simulink model "anti_windup_cliping_back_calculation"  (R2022b)
settings: Solver=FixedStepAuto  StartTime=0.0  StopTime=200  FixedStep=0.001  RelTol=1e-3
libraries: simulink x2
settings Model: Creator=mrxmi  LastModifiedBy=mrxmi

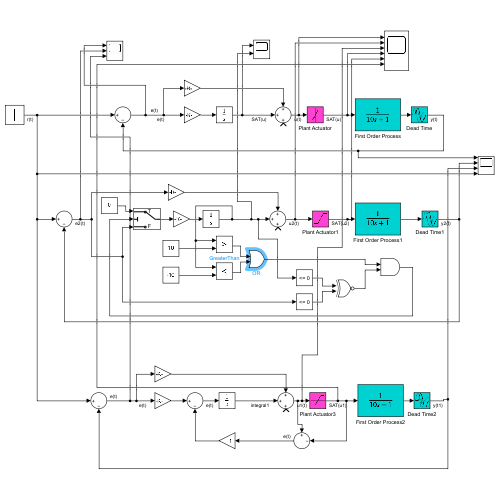
[thumbnail: Simulink's stored preview of the top-level diagram]
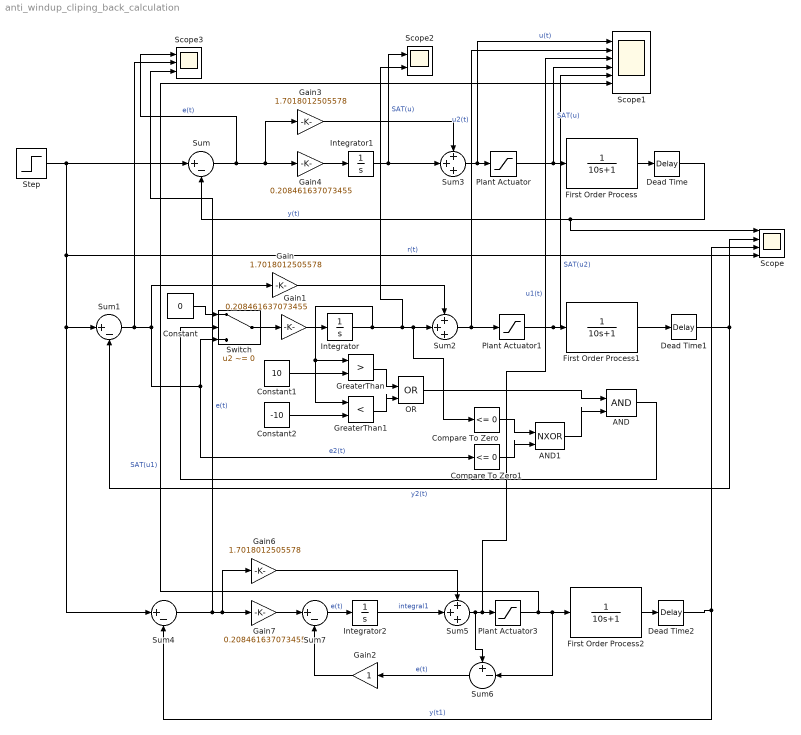
== system anti_windup_cliping_back_calculation ==
  AND : Logic  IconShape=distinctive  AllPortsSameDT=off  OutDataTypeStr=boolean
  AND1 : Logic  Operator=NXOR  IconShape=distinctive  AllPortsSameDT=off  OutDataTypeStr=boolean
  Compare To Zero : simulink/Logic and Bit Operations/Compare To Zero  relop=<=  OutDataTypeStr=boolean
  Compare To Zero1 : simulink/Logic and Bit Operations/Compare To Zero  relop=<=  OutDataTypeStr=boolean
  Constant : Constant  Value=0
  Constant1 : Constant  Value=10
  Constant2 : Constant  Value=-10
  Dead Time : TransportDelay  DelayTime=2  BufferSize=2048
  Dead Time1 : TransportDelay  DelayTime=2  BufferSize=2048
  Dead Time2 : TransportDelay  DelayTime=2  BufferSize=2048
  First Order Process : TransferFcn  Numerator=1  Denominator=[10 1]
  First Order Process1 : TransferFcn  Numerator=1  Denominator=[10 1]
  First Order Process2 : TransferFcn  Numerator=1  Denominator=[10 1]
  Gain : Gain  Gain=1.7018012505578
  Gain1 : Gain  Gain=0.208461637073455
  Gain2 : Gain
  Gain3 : Gain  Gain=1.7018012505578
  Gain4 : Gain  Gain=0.208461637073455
  Gain6 : Gain  Gain=1.7018012505578
  Gain7 : Gain  Gain=0.208461637073455
  GreaterThan : RelationalOperator  Operator=>  OutDataTypeStr=boolean  RndMeth=Simplest  InputSameDT=off
  GreaterThan1 : RelationalOperator  Operator=<  OutDataTypeStr=boolean  RndMeth=Simplest  InputSameDT=off
  Integrator : Integrator
  Integrator1 : Integrator
  Integrator2 : Integrator
  OR : Logic  Operator=OR  IconShape=distinctive  AllPortsSameDT=off  OutDataTypeStr=boolean
  Plant Actuator : Saturate  UpperLimit=10  LowerLimit=-10
  Plant Actuator1 : Saturate  UpperLimit=10  LowerLimit=-10
  Plant Actuator3 : Saturate  UpperLimit=10  LowerLimit=-10
  Scope : Scope  NumInputPorts=4
  Scope1 : Scope  NumInputPorts=6
  Scope2 : Scope  NumInputPorts=2
  Scope3 : Scope  NumInputPorts=3
  Step : Step  Time=80  Before=10  After=5  SampleTime=0
  Sum{,1,4,7} (4 alike) : Sum  Inputs=|+-
  Sum2 : Sum  Inputs=+++
  Sum3 : Sum  Inputs=+++
  Sum5 : Sum  Inputs=+++
  Sum6 : Sum  Inputs=+-|
  Switch : Switch  Criteria=u2 ~= 0  SaturateOnIntegerOverflow=off  InputSameDT=off
  wires:
  Dead Time/1 -> Scope/1, Sum/2  "y(t)"
  Plant Actuator/1 -> Scope1/4, First Order Process/1  "SAT(u)"
  Step/1 -> Scope/4, Sum4/1, Sum1/1, Sum/1  "r(t)"
  First Order Process/1 -> Dead Time/1
  Gain1/1 -> Integrator/1
  Gain/1 -> Sum2/1
  Sum1/1 -> Scope3/2, Compare To Zero1/1, Switch/3, Gain/1  "e2(t)"
  Sum2/1 -> Plant Actuator1/1, Scope1/2  "u2(t)"
  Plant Actuator1/1 -> Scope1/5, First Order Process1/1  "SAT(u2)"
  First Order Process1/1 -> Dead Time1/1
  Dead Time1/1 -> Sum1/2, Scope/2  "y2(t)"
  Integrator/1 -> GreaterThan/1, GreaterThan1/1, Compare To Zero/1, Sum2/2, Scope2/2
  Integrator1/1 -> Scope2/1, Sum3/2  "SAT(u)"
  Sum/1 -> Scope3/1, Gain4/1, Gain3/1  "e(t)"
  Gain3/1 -> Sum3/1
  Gain4/1 -> Integrator1/1
  Sum3/1 -> Scope1/1, Plant Actuator/1  "u(t)"
  Integrator2/1 -> Sum5/2  "integral1"
  Gain6/1 -> Sum5/1
  Sum4/1 -> Scope3/3, Gain7/1, Gain6/1  "e(t)"
  Dead Time2/1 -> Sum4/2, Scope/3  "y(t1)"
  Plant Actuator3/1 -> Scope1/6, Sum6/2, First Order Process2/1  "SAT(u1)"
  First Order Process2/1 -> Dead Time2/1
  Sum5/1 -> Scope1/3, Plant Actuator3/1, Sum6/1  "u1(t)"
  Switch/1 -> Gain1/1
  Constant/1 -> Switch/1
  GreaterThan/1 -> OR/1
  Constant1/1 -> GreaterThan/2
  Constant2/1 -> GreaterThan1/2
  GreaterThan1/1 -> OR/2
  OR/1 -> AND/1
  AND/1 -> Switch/2
  AND1/1 -> AND/2
  Compare To Zero1/1 -> AND1/2
  Compare To Zero/1 -> AND1/1
  Sum6/1 -> Gain2/1  "e(t)"
  Gain7/1 -> Sum7/1
  Sum7/1 -> Integrator2/1  "e(t)"
  Gain2/1 -> Sum7/2
